simulink model "dtc_svpwm"  (Simulink 8.6)
settings: Solver=ode45  StartTime=0.0  StopTime=0.1  MaxStep=0.00001  RelTol=1e-3
libraries: powerlib x5, powerlib_extras x1
settings Model: Creator=Administrator  LastModifiedBy=Administrator
settings SolverCC: ZeroCrossControl=DisableAll
settings OptimizationCC: InitFltsAndDblsToZero=on
settings DebuggingCC: FcnCallInpInsideContextMsg=UseLocalSettings
settings GRTTargetCC: GeneratePreprocessorConditionals=Use local settings

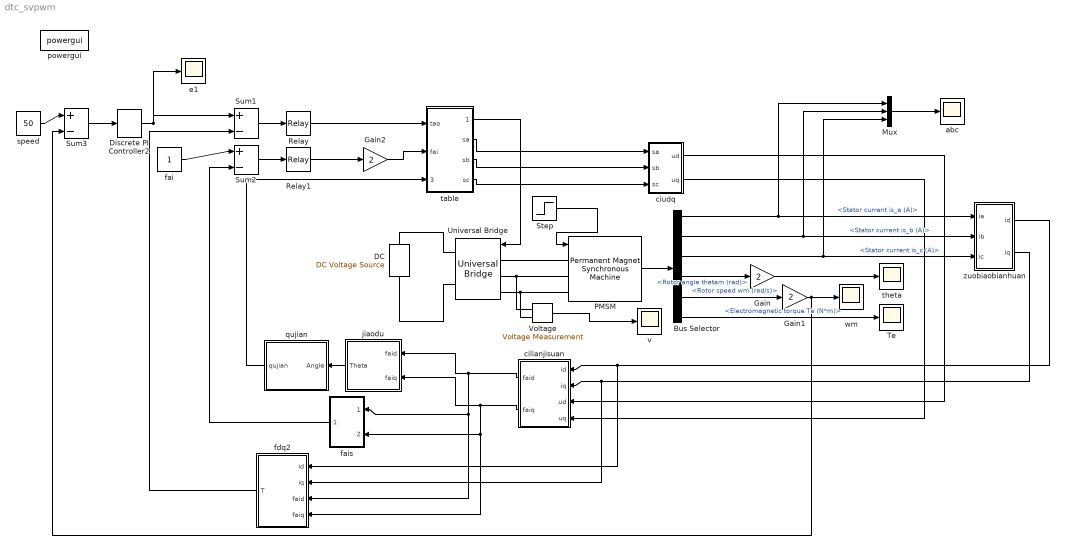
== system dtc_svpwm ==
  Bus Selector : BusSelector  OutputSignals=Stator current is_a (A),Stator current is_b (A),Stator current is_c (A),Rotor angle thetam (rad),Rotor speed wm (rad/s),Electromagnetic torque Te (N*m)
  "DC " : powerlib/Electrical Sources/DC Voltage Source  Amplitude=310  Measurements=None
  Discrete PI Controller2 : powerlib_extras/Discrete  Control Blocks/Discrete PI Controller  Kp=0.5  Ki=2  Par_Limits=[3 -3]  Init=0  Ts=1e-4
  Gain : Gain  Gain=2
  Gain1 : Gain  Gain=2
  Gain2 : Gain  Gain=2
  Mux : Mux  Inputs=3
  PMSM : powerlib/Machines/Permanent Magnet Synchronous Machine  NbPhases=3  FluxDistribution=Sinusoidal  RotorType=Round  MechanicalLoad=Torque Tm  PresetModel=No  ShowDetailedParameters=on  MeasurementBus=off  Resistance=3  Inductance=8.5e-3  dqInductances=[0.168;0.168]  La=0.000395  MachineConstant=Flux linkage established by magnets (V.s)  Flux=0.175  VoltageCst=63.483  TorqueCst=0.525  Flat=120  Mechanical=[0.008 0 2]  PolePairs=2  InitialConditions=[0,0, 0,0]  InitialConditions5ph=[0 0 0 0 0 0]  TsPowergui=0  TsBlock=-1  RefAngle=90 degrees behind phase A axis (modified Park)
  Relay : Relay  OnSwitchValue=0.05  OffSwitchValue=-0.05
  Relay1 : Relay  OnSwitchValue=0.005  OffSwitchValue=-0.005
  Step : Step  Time=0.01  Before=1  After=2  SampleTime=0
  Sum1 : Sum  Inputs=|+-
  Sum2 : Sum  Inputs=|+-
  Sum3 : Sum  Inputs=|+-
  Te : Scope
  Universal Bridge : powerlib/Power Electronics/Universal Bridge  Arms=3  SnubberResistance=1e5  SnubberCapacitance=inf  Device=IGBT / Diodes  Ron=1e-3  Lon=0  ForwardVoltages="[  0  0  ]"  ForwardVoltage=0  GTOparameters=[ 10e-6 , 20e-6 ]  IGBTparameters=[ 1e-6 , 2e-6 ]  Measurements=None  Measurements_2=None  converterType=Rectifier
  "Voltage " : powerlib/Measurements/Voltage Measurement  PhasorSimulation=off  OutputType=Complex  PSBequivalent=0
  abc : Scope
  cilianjisuan : Subsystem
  ciudq : Subsystem
  e1 : Scope
  fai : Constant
  fais : Subsystem
  fdq2 : Subsystem
  jiaodu : Subsystem
  powergui : powerlib/powergui  SimulationMode=Continuous  SolverType=Tustin/Backward Euler (TBE)  SampleTime=50e-6  frequency=60  SPID=off  DisableSnubberDevices=off  DisableRonSwitches=off  DisableVfSwitches=off  SwTol=0  DisplayEquations=off  Interpol=off  ExternalGateDelay=off  methode=off  Ts=0  FunctionMessages=off  echomessages=off  HookPort=off  EnableUseOfTLC=off  x0status=blocks  frequencyindice=0  Pbase=100e6  ErrMax=1e-4  Iterations=50  UnitsV=kV  UnitsW=MW  buscounter=0  RestoreLinks=warning  ResistiveCurrentMeasurement=off  Frange=[0:2:500]  Ylog=off  Xlog=on  ShowGrid=off  save=off  variable=ZData  structure=0  ZoomFFT=on  StartTime=0.0  cycles=1  DisplayStyle=1  fundamental=60  FreqAxis=off  MaxFrequency=1000  frequencyindicesteady=1  RmsSteady=1  display=off
  qujian : Subsystem
  speed : Constant  Value=50
  table : Subsystem
  theta : Scope
  v : Scope
  wm : Scope
  zuobiaobianhuan : Subsystem  mask(bianhuan){}
  wires:
  table/1(Pulse) -> Universal Bridge/1
  PMSM/1 -> Bus Selector/1
  Bus Selector/4 -> Gain/1  "<Rotor angle thetam (rad)>"
  Gain/1 -> theta/1
  Bus Selector/6 -> Te/1  "<Electromagnetic torque Te (N*m)>"
  Gain1/1 -> wm/1, Sum3/2
  Step/1 -> PMSM/1
  Sum1/1 -> Relay/1
  Sum2/1 -> Relay1/1
  fais/1(fais) -> Sum2/2
  fai/1 -> Sum2/1
  fdq2/1(T) -> Sum1/2
  jiaodu/1(Theta) -> qujian/1(Angle)
  cilianjisuan/1(faid) -> jiaodu/1(faid), fdq2/3(faid), fais/1(faid)
  cilianjisuan/2(faiq) -> jiaodu/2(faiq), fdq2/4(faiq), fais/2(faiq)
  table/3(sb) -> ciudq/2(sb)
  speed/1 -> Sum3/1
  Bus Selector/5 -> Gain1/1  "<Rotor speed wm (rad/s)>"
  table/2(sa) -> ciudq/1(sa)
  table/4(sc) -> ciudq/3(sc)
  zuobiaobianhuan/1(id) -> fdq2/1(id), cilianjisuan/1(id)
  zuobiaobianhuan/2(iq) -> fdq2/2(iq), cilianjisuan/2(iq)
  Bus Selector/1 -> zuobiaobianhuan/1(ia), Mux/1  "<Stator current is_a (A)>"
  Bus Selector/2 -> zuobiaobianhuan/2(ib), Mux/2  "<Stator current is_b (A)>"
  Bus Selector/3 -> zuobiaobianhuan/3(ic), Mux/3  "<Stator current is_c (A)>"
  Relay/1 -> table/1(tao)
  qujian/1(qujian) -> table/3(theta)
  Sum3/1 -> Discrete PI Controller2/1
  Discrete PI Controller2/1 -> Sum1/1, e1/1
  ciudq/1(ud) -> cilianjisuan/3(ud)
  ciudq/2(uq) -> cilianjisuan/4(uq)
  Relay1/1 -> Gain2/1
  Gain2/1 -> table/2(fai)
  "Voltage "/1 -> v/1
  Mux/1 -> abc/1
  connections:
  "DC "/RConn1 -- Universal Bridge/RConn1
  "DC "/LConn1 -- Universal Bridge/RConn2
  Universal Bridge/LConn1 -- PMSM/LConn1
  Universal Bridge/LConn2 -- PMSM/LConn2 -- "Voltage "/LConn1
  Universal Bridge/LConn3 -- PMSM/LConn3 -- "Voltage "/LConn2

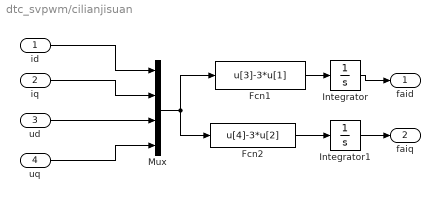
== system dtc_svpwm/cilianjisuan ==
  id : Inport
  iq : Inport  Port=2
  ud : Inport  Port=3
  uq : Inport  Port=4
  Fcn1 : Fcn  Expr=u[3]-3*u[1]
  Fcn2 : Fcn  Expr=u[4]-3*u[2]
  Integrator : Integrator  InitialCondition=0.01
  Integrator1 : Integrator  InitialCondition=0.01
  Mux : Mux
  faid : Outport
  faiq : Outport  Port=2
  wires:
  id/1 -> Mux/1
  iq/1 -> Mux/2
  ud/1 -> Mux/3
  uq/1 -> Mux/4
  Mux/1 -> Fcn1/1, Fcn2/1
  Integrator/1 -> faid/1
  Fcn1/1 -> Integrator/1
  Integrator1/1 -> faiq/1
  Fcn2/1 -> Integrator1/1

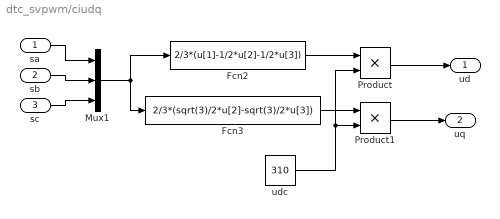
== system dtc_svpwm/ciudq ==
  sa : Inport
  sb : Inport  Port=2
  sc : Inport  Port=3
  Fcn2 : Fcn  Expr=2/3*(u[1]-1/2*u[2]-1/2*u[3])
  Fcn3 : Fcn  Expr=2/3*(sqrt(3)/2*u[2]-sqrt(3)/2*u[3])
  Mux1 : Mux  Inputs=3
  Product : Product  RndMeth=Zero
  Product1 : Product  RndMeth=Zero
  udc : Constant  Value=310
  ud : Outport
  uq : Outport  Port=2
  wires:
  sa/1 -> Mux1/1
  sb/1 -> Mux1/2
  sc/1 -> Mux1/3
  Mux1/1 -> Fcn2/1, Fcn3/1
  Fcn2/1 -> Product/1
  udc/1 -> Product/2, Product1/2
  Fcn3/1 -> Product1/1
  Product/1 -> ud/1
  Product1/1 -> uq/1

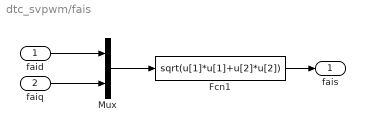
== system dtc_svpwm/fais ==
  faid : Inport
  faiq : Inport  Port=2
  Fcn1 : Fcn  Expr=sqrt(u[1]*u[1]+u[2]*u[2])
  Mux : Mux  Inputs=2
  fais : Outport
  wires:
  faid/1 -> Mux/1
  faiq/1 -> Mux/2
  Mux/1 -> Fcn1/1
  Fcn1/1 -> fais/1

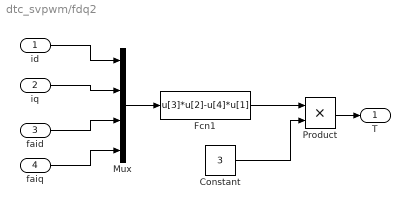
== system dtc_svpwm/fdq2 ==
  id : Inport
  iq : Inport  Port=2
  faid : Inport  Port=3
  faiq : Inport  Port=4
  Constant : Constant  Value=3
  Fcn1 : Fcn  Expr=u[3]*u[2]-u[4]*u[1]
  Mux : Mux
  Product : Product  RndMeth=Zero
  T : Outport
  wires:
  id/1 -> Mux/1
  iq/1 -> Mux/2
  faid/1 -> Mux/3
  faiq/1 -> Mux/4
  Mux/1 -> Fcn1/1
  Fcn1/1 -> Product/1
  Constant/1 -> Product/2
  Product/1 -> T/1

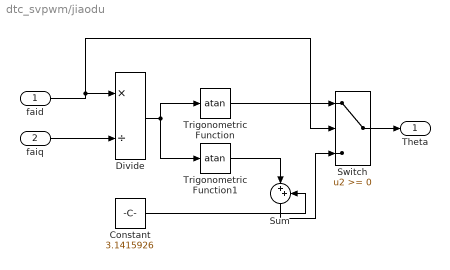
== system dtc_svpwm/jiaodu ==
  faid : Inport
  faiq : Inport  Port=2
  Constant : Constant  Value=3.1415926
  Divide : Product  Inputs=*/
  Sum : Sum  Inputs=|++
  Switch : Switch
  Trigonometric Function : Trigonometry  Operator=atan
  Trigonometric Function1 : Trigonometry  Operator=atan
  Theta : Outport
  wires:
  faid/1 -> Divide/1, Switch/2
  faiq/1 -> Divide/2
  Trigonometric Function/1 -> Switch/1
  Sum/1 -> Switch/3
  Constant/1 -> Sum/2
  Switch/1 -> Theta/1
  Divide/1 -> Trigonometric Function1/1, Trigonometric Function/1
  Trigonometric Function1/1 -> Sum/1

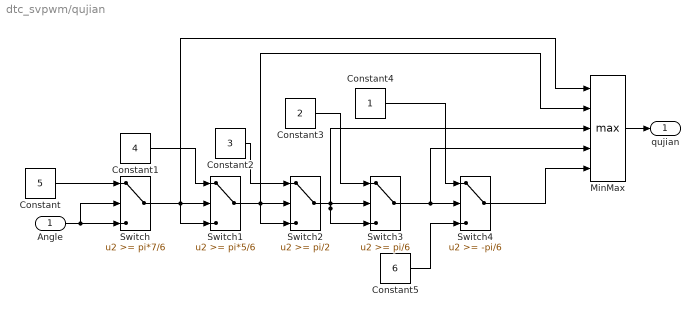
== system dtc_svpwm/qujian ==
  Angle : Inport
  Constant : Constant  Value=5
  Constant1 : Constant  Value=4
  Constant2 : Constant  Value=3
  Constant3 : Constant  Value=2
  Constant4 : Constant
  Constant5 : Constant  Value=6
  MinMax : MinMax  Function=max  Inputs=5
  Switch : Switch  Threshold=pi*7/6
  Switch1 : Switch  Threshold=pi*5/6
  Switch2 : Switch  Threshold=pi/2
  Switch3 : Switch  Threshold=pi/6
  Switch4 : Switch  Threshold=-pi/6
  qujian : Outport
  wires:
  Angle/1 -> Switch/3, Switch/2
  Constant/1 -> Switch/1
  Switch/1 -> Switch1/2, Switch1/3, MinMax/1
  Switch1/1 -> MinMax/2, Switch2/2, Switch2/3
  Constant1/1 -> Switch1/1
  Constant2/1 -> Switch2/1
  Constant3/1 -> Switch3/1
  Switch4/1 -> MinMax/5
  Constant4/1 -> Switch4/1
  MinMax/1 -> qujian/1
  Constant5/1 -> Switch4/3
  Switch2/1 -> Switch3/2, Switch3/3, MinMax/3
  Switch3/1 -> Switch4/2, MinMax/4

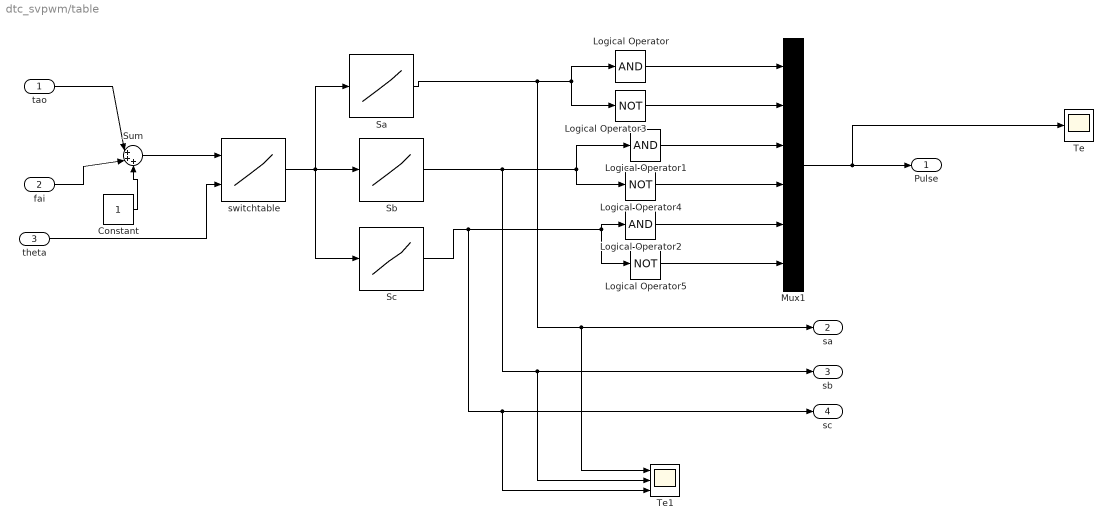
== system dtc_svpwm/table ==
  tao : Inport
  fai : Inport  Port=2
  theta : Inport  Port=3
  Constant : Constant
  Logical Operator : Logic  Inputs=1  AllPortsSameDT=off  OutDataTypeStr=boolean
  Logical Operator1 : Logic  Inputs=1  AllPortsSameDT=off  OutDataTypeStr=boolean
  Logical Operator2 : Logic  Inputs=1  AllPortsSameDT=off  OutDataTypeStr=boolean
  Logical Operator3 : Logic  Operator=NOT  Inputs=1  AllPortsSameDT=off  OutDataTypeStr=boolean
  Logical Operator4 : Logic  Operator=NOT  Inputs=1  AllPortsSameDT=off  OutDataTypeStr=boolean
  Logical Operator5 : Logic  Operator=NOT  Inputs=1  AllPortsSameDT=off  OutDataTypeStr=boolean
  Mux1 : Mux  Inputs=6
  Sa : Lookup_n-D  NumberOfTableDimensions=1  BreakpointsForDimension1=[1:6]  Table="[1 1  0 0 0 1]"  InputSameDT=on
  Sb : Lookup_n-D  NumberOfTableDimensions=1  BreakpointsForDimension1=[1:6]  Table=[0 1 1 1 0 0]  InputSameDT=on
  Sc : Lookup_n-D  NumberOfTableDimensions=1  BreakpointsForDimension1=[1,2,3,4,5,6]  Table=[0,0,0,1,1,1]  InputSameDT=on
  Sum : Sum  Inputs=|+++
  Te : Scope
  Te1 : Scope  NumInputPorts=3
  switchtable : Lookup_n-D  BreakpointsForDimension1=[1:4]  BreakpointsForDimension2=[1:6]  Table=[2 3 4 5 6 1;6 1 2 3 4 5 ;3 4 5 6 1 2;5 6 1 2 3 4]  InputSameDT=on
  Pulse : Outport
  sa : Outport  Port=2
  sb : Outport  Port=3
  sc : Outport  Port=4
  wires:
  switchtable/1 -> Sa/1, Sc/1, Sb/1
  theta/1 -> switchtable/2
  Sb/1 -> Logical Operator1/1, Logical Operator4/1, sb/1, Te1/2
  Sc/1 -> Logical Operator2/1, Logical Operator5/1, sc/1, Te1/3
  Sa/1 -> Logical Operator/1, Logical Operator3/1, sa/1, Te1/1
  Logical Operator3/1 -> Mux1/2
  Logical Operator4/1 -> Mux1/4
  Logical Operator5/1 -> Mux1/6
  Mux1/1 -> Pulse/1, Te/1
  Logical Operator/1 -> Mux1/1
  Logical Operator1/1 -> Mux1/3
  Logical Operator2/1 -> Mux1/5
  Constant/1 -> Sum/3
  Sum/1 -> switchtable/1
  fai/1 -> Sum/2
  tao/1 -> Sum/1

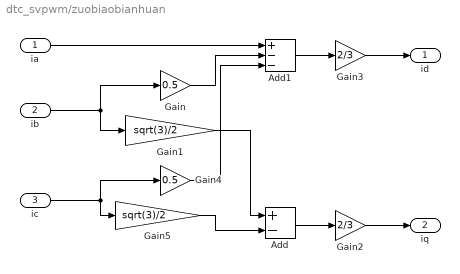
== system dtc_svpwm/zuobiaobianhuan ==
  ia : Inport
  ib : Inport  Port=2
  ic : Inport  Port=3
  Add : Sum  Inputs=+-
  Add1 : Sum  Inputs=+--
  Gain : Gain  Gain=0.5
  Gain1 : Gain  Gain=sqrt(3)/2
  Gain2 : Gain  Gain=2/3
  Gain3 : Gain  Gain=2/3
  Gain4 : Gain  Gain=0.5
  Gain5 : Gain  Gain=sqrt(3)/2
  id : Outport
  iq : Outport  Port=2
  wires:
  ic/1 -> Gain5/1, Gain4/1
  ib/1 -> Gain1/1, Gain/1
  Gain1/1 -> Add/1
  Gain4/1 -> Add1/3
  Gain/1 -> Add1/2
  ia/1 -> Add1/1
  Gain5/1 -> Add/2
  Gain3/1 -> id/1
  Gain2/1 -> iq/1
  Add/1 -> Gain2/1
  Add1/1 -> Gain3/1
